simulink model "IMU_euler_angles_and_rates_with_checksum"  (Simulink 7.8)
settings: Solver=ode45  StartTime=0.0  StopTime=10.0  RelTol=1e-3
undefined symbols (not defined in the file or in its folder): Com1, none
libraries: xpcseriallib x2, xpclib x2
settings Model: Creator=kevinsg  LastModifiedBy=kevinsg

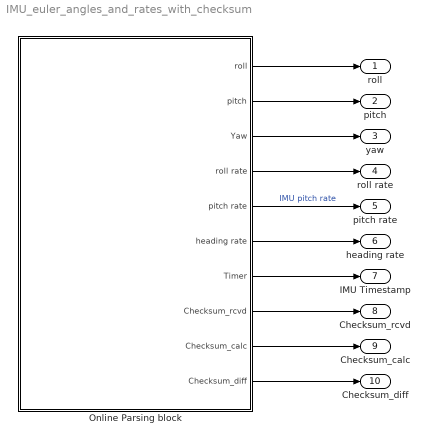
== system IMU_euler_angles_and_rates_with_checksum ==
  Online Parsing block : Subsystem
  roll : Outport
  pitch : Outport  Port=2
  yaw : Outport  Port=3
  roll rate : Outport  Port=4
  pitch rate : Outport  Port=5
  heading rate : Outport  Port=6
  IMU Timestamp : Outport  Port=7
  Checksum_rcvd : Outport  Port=8
  Checksum_calc : Outport  Port=9
  Checksum_diff : Outport  Port=10
  wires:
  Online Parsing block/1(roll) -> roll/1
  Online Parsing block/2(pitch) -> pitch/1
  Online Parsing block/3(Yaw) -> yaw/1
  Online Parsing block/4(roll rate) -> roll rate/1
  Online Parsing block/5(pitch rate) -> pitch rate/1  "IMU pitch rate"
  Online Parsing block/6(heading rate) -> heading rate/1
  Online Parsing block/7(Timer) -> IMU Timestamp/1
  Online Parsing block/8(Checksum_rcvd) -> Checksum_rcvd/1
  Online Parsing block/9(Checksum_calc) -> Checksum_calc/1
  Online Parsing block/10(Checksum_diff) -> Checksum_diff/1

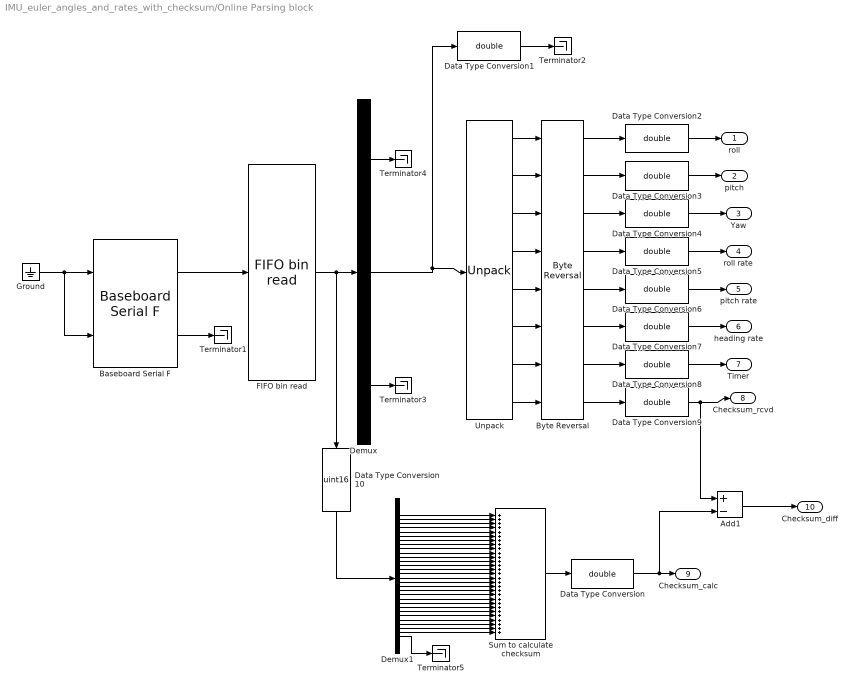
== system IMU_euler_angles_and_rates_with_checksum/Online Parsing block ==
  Add1 : Sum  Inputs=+-
  Baseboard Serial F : xpcseriallib/Mainboard/Baseboard Serial F  group=Basic Setup  port=1  irqnum=4  saddr1=0x3f8  saddr2=0x3e8  config=Com1/none  baud1=115200  parity1=None  ndata1=8  nstop1=1  fifomode1=64 deep  rlevel1=almost full  automode1=off  xmtfifosize1=1024  xmtdatatype1=8 bit uint null terminated  rcvfifosize1=1024  baud2=115200  parity2=None  ndata2=8  nstop2=1  fifomode2=16 deep  rlevel2=half full  automode2=off  xmtfifosize2=1024  xmtdatatype2=8 bit uint null terminated  rcvfifosize2=1024
  Byte Reversal : xpclib/UDP/Byte Reversal  numInp=8
  Data Type Conversion{,1..9} (10 alike) : DataTypeConversion  OutDataTypeStr=double
  Data Type Conversion10 : DataTypeConversion  OutDataTypeStr=uint16
  Demux : Demux  Outputs=[1 30 -1]
  Demux1 : Demux  Outputs=[1 1 1 1 1 1 1 1 1 1 1 1 1 1 1 1 1 1 1 1 1 1 1 1 1 1 1 1 1 -1]
  "FIFO bin read " : xpcseriallib/FIFO bin read   header={uint8([207])}  lengths=[31]  hold=Hold last output if no new data  enable=off  maxsize=32  outputtype=8 bit uint null terminated  sampletime=0.001
  Ground : Ground
  Sum to calculate checksum : Sum  Inputs=29
  Terminator{1..5} (5 alike) : Terminator
  Unpack : xpclib/UDP/Unpack  dimensions={[1],[1],[1],[1],[1],[1],[1],[1]}  datatypes={'single','single','single','single','single','single','uint32','uint16'}  byteAlign=1
  roll : Outport
  pitch : Outport  Port=2
  Yaw : Outport  Port=3
  roll rate : Outport  Port=4
  pitch rate : Outport  Port=5
  heading rate : Outport  Port=6
  Timer : Outport  Port=7
  Checksum_rcvd : Outport  Port=8
  Checksum_calc : Outport  Port=9
  Checksum_diff : Outport  Port=10
  wires:
  Ground/1 -> Baseboard Serial F/1, Baseboard Serial F/2
  Baseboard Serial F/1 -> "FIFO bin read "/1
  Baseboard Serial F/2 -> Terminator1/1
  "FIFO bin read "/1 -> Demux/1, Data Type Conversion10/1
  Demux/3 -> Terminator3/1
  Demux/2 -> Data Type Conversion1/1, Unpack/1
  Demux/1 -> Terminator4/1
  Data Type Conversion1/1 -> Terminator2/1
  Unpack/1 -> Byte Reversal/1
  Unpack/2 -> Byte Reversal/2
  Unpack/3 -> Byte Reversal/3
  Unpack/4 -> Byte Reversal/4
  Unpack/5 -> Byte Reversal/5
  Unpack/6 -> Byte Reversal/6
  Unpack/7 -> Byte Reversal/7
  Unpack/8 -> Byte Reversal/8
  Data Type Conversion2/1 -> roll/1
  Data Type Conversion3/1 -> pitch/1
  Data Type Conversion4/1 -> Yaw/1
  Data Type Conversion5/1 -> roll rate/1
  Data Type Conversion6/1 -> pitch rate/1
  Data Type Conversion7/1 -> heading rate/1
  Data Type Conversion8/1 -> Timer/1
  Byte Reversal/1 -> Data Type Conversion2/1
  Byte Reversal/2 -> Data Type Conversion3/1
  Byte Reversal/3 -> Data Type Conversion4/1
  Byte Reversal/4 -> Data Type Conversion5/1
  Byte Reversal/5 -> Data Type Conversion6/1
  Byte Reversal/6 -> Data Type Conversion7/1
  Byte Reversal/7 -> Data Type Conversion8/1
  Demux1/30 -> Terminator5/1
  Demux1/1 -> Sum to calculate checksum/1
  Demux1/2 -> Sum to calculate checksum/2
  Demux1/3 -> Sum to calculate checksum/3
  Demux1/4 -> Sum to calculate checksum/4
  Demux1/5 -> Sum to calculate checksum/5
  Demux1/6 -> Sum to calculate checksum/6
  Demux1/7 -> Sum to calculate checksum/7
  Demux1/8 -> Sum to calculate checksum/8
  Demux1/9 -> Sum to calculate checksum/9
  Demux1/10 -> Sum to calculate checksum/10
  Demux1/11 -> Sum to calculate checksum/11
  Demux1/12 -> Sum to calculate checksum/12
  Demux1/13 -> Sum to calculate checksum/13
  Demux1/14 -> Sum to calculate checksum/14
  Demux1/15 -> Sum to calculate checksum/15
  Demux1/16 -> Sum to calculate checksum/16
  Demux1/17 -> Sum to calculate checksum/17
  Demux1/18 -> Sum to calculate checksum/18
  Demux1/19 -> Sum to calculate checksum/19
  Demux1/20 -> Sum to calculate checksum/20
  Demux1/21 -> Sum to calculate checksum/21
  Demux1/22 -> Sum to calculate checksum/22
  Demux1/23 -> Sum to calculate checksum/23
  Demux1/24 -> Sum to calculate checksum/24
  Demux1/25 -> Sum to calculate checksum/25
  Demux1/26 -> Sum to calculate checksum/26
  Demux1/27 -> Sum to calculate checksum/27
  Demux1/28 -> Sum to calculate checksum/28
  Demux1/29 -> Sum to calculate checksum/29
  Data Type Conversion9/1 -> Checksum_rcvd/1, Add1/1
  Byte Reversal/8 -> Data Type Conversion9/1
  Sum to calculate checksum/1 -> Data Type Conversion/1
  Data Type Conversion/1 -> Checksum_calc/1, Add1/2
  Data Type Conversion10/1 -> Demux1/1
  Add1/1 -> Checksum_diff/1
